simulink model "RT_01"  (R2018b)
settings: Solver=FixedStepAuto  StartTime=0.0  StopTime=40  FixedStep=0.01  RelTol=1e-3
undefined symbols (not defined in the file): circle, DiscIntNeverNeededParam, Measurement_Computing, National_Instruments, PCI, QUAD04
libraries: sldrtlib x25, simulink x8, simulink_extras x2
(part 2 of 2)

== matlab function RT_01/Set point/Path Planning Circle/Inverse Kinematics JS1 ==
  data: EE_r input; P output; solution input
function P  = IK_JS(EE_r,solution)
a1=75; a2=270; a3=90; d1=335; d4=295; d7=80;
l = size(EE_r,1);   % Số điểm cần tính động học nghịch khi quy hoạch đường đi
emt1 = zeros(l,13); % Mảng rỗng để chứa ngõ t, the(t), v(t)
for n=1:l           % Vòng for tính động học nghịch từng điểm
    emt = zeros(8,6);
    m = 0;
    px =    EE_r(n,2);
    py =    EE_r(n,3);
    pz =    EE_r(n,4);
    roll =  EE_r(n,5);  
    pitch = EE_r(n,6);
    yaw =   EE_r(n,7);
    r11 = cos(yaw)*cos(pitch);
    r21 = sin(yaw)*cos(pitch);
    r31 = -sin(pitch);
    r12 = cos(yaw)*sin(pitch)*sin(roll) - sin(yaw)*cos(roll);
    r22 = sin(yaw)*sin(pitch)*sin(roll) + cos(yaw)*cos(roll);
    r32 = cos(pitch)*sin(roll);
    r13 = cos(yaw)*sin(pitch)*cos(roll) + sin(yaw)*sin(roll);
    r23 = sin(yaw)*sin(pitch)*cos(roll) - cos(yaw)*sin(roll);
    r33 = cos(pitch)*cos(roll);
    % Find the1
    a_1 = py - r23*d7;
    b_1 = - px + r13*d7;
    d_1 = 0;
    the11 = basic_01(a_1,b_1,d_1);

    for i = 1:2
        % Find the2
        u = cos(the11(i))*(px-d7*r13) + sin(the11(i))*(py-r23*d7) - a1;
        v = pz - d1 - r33*d7;
        a_2 = v;
        b_2 = u;
        d_2 = (a3^2+d4^2-u^2-v^2-a2^2)/(-2*a2);
        if a_2*a_2 + b_2*b_2 - d_2*d_2 >=0
            the22 = basic_01(a_2,b_2,d_2);
        else
            continue;
        end

        for j = 1:2
            % Find the3
            a_3 = a3;
            b_3 = d4;
            c_3 = u*sin(the22(j)) + v*cos(the22(j)) - a2;
            d_3 = u*cos(the22(j)) - v*sin(the22(j));
            the33 = basic_02(a_3,b_3,c_3,d_3);

            % Find the5
            c5 = (r13*cos(the11(i))*cos(the22(j)) - r33*sin(the22(j)) + r23*cos(the22(j))*sin(the11(i)))*cos(the33) - (r33*cos(the22(j)) + r13*cos(the11(i))*sin(the22(j)) + r23*sin(the11(i))*sin(the22(j)))*sin(the33);
            if 1*1 + 0*0 - c5*c5 >=0
                the55 = basic_01(1,0,c5);
            else
                continue;
            end
            for k = 1:2
                % Find the4
                m = m+1;
                s4 = (r23*cos(the11(i)) - r13*sin(the11(i)))/(sin(the55(k)));
                c4 = (r33*cos(the22(j)) + r13*cos(the11(i))*sin(the22(j)) + r23*sin(the11(i))*sin(the22(j)) + sin(the33)*cos(the55(k))) / (-cos(the33)*sin(the55(k)));
                the44 = atan2(s4,c4);

                % Find the6
                a_6 = r21*cos(the11(i)) - r11*sin(the11(i));
                b_6 = r22*cos(the11(i)) - r12*sin(the11(i));
                c_6 = -sin(the44)*cos(the55(k));
                d_6 = cos(the44);
                the66 = basic_02(a_6,b_6,c_6,-d_6);
                emt(m,:)=[the11(i),the22(j),the33,the44,the55(k),the66];
            end
        end
    end
    % the = emt(solution,:);
    the1 = emt(solution,1);
    the2 = emt(solution,2);
    the3 = emt(solution,3);
    the4 = emt(solution,4);
    the5 = emt(solution,5);
    the6 = emt(solution,6);
%     the_r = [the1;the2;the3;the4;the5;the6];
%     emt1(n,:) = [(n-1)*t/l,the1,the2,the3,the4,the5,the6,0,0,0,0,0,0];
    emt1(n,:) = [EE_r(n,1),the1,the2,the3,the4,the5,the6,0,0,0,0,0,0];
end
P=emt1;
end

function x = basic_01(a, b, d) % a*cos(x) + b*sin(x) = d
    anp = atan2(b, a);
    
    x1 = anp + atan2(sqrt(a*a + b*b - d*d), d);
    x2 = anp + atan2(-sqrt(a*a + b*b - d*d), d);
    x = [x1; x2];
end   

function x = basic_02(a, b, c, d) 
    % a*cos(x) - b*sin(x) = c
    % b*cos(x) + a*sin(x) = d
    sin = (d - b*c/a) / (b^2/a + a);
    cos = (c + b*d/a) / (b^2/a + a);
    x = atan2(sin,cos);
end

== matlab function RT_01/Set point/Path Planning Circle/Circle CS ==
  data: clock input; EE_r output
function EE_r = TP_Circle(clock)
% H=ScopeData.signals.values(:,1:3);
t = clock-10;
f=0.1; %hz
Px_r = 450;
Py_r = 0+100*sin(2*pi*f*t);
Pz_r = 550+100*cos(2*pi*f*t);
% roll_r=pi/3;
% pitch_r=pi/6;
% yaw_r=pi/2;
roll_r = 0*pi/2;
pitch_r = -pi/2;
yaw_r = pi;
EE_r = [Px_r,Py_r,Pz_r,roll_r,pitch_r,yaw_r]';

== matlab function RT_01/Set point/Path Planning Circle/Trajectory Planning CS ==
  data: clock input; EE_r output; P input
function EE_r = TP_CS_6DOF(clock,P)
t=clock;
% H=ScopeData.signals.values(:,1:3); Lưu data để sử dụng spline
%% Quy hoạch quỹ đạo
k = size(P,1)-1;                    % Số giai đoạn chạy, i điểm thì i-1 giai đoạn
ai = zeros(k,24);                    % Ma trận K*8 lưu các giá trị a0 - a4 của X, Y
for i=1:k
    ai(i,:) = TP_CS(P(i,:),P(i+1,:));  % Tính giá trị a0 - a4 đối với từng điểm P(x,y)
end
%% Xuất quỹ đạo
% P0 = [ti; q0x; q0y; q0z; q0roll; q0pitch; q0yaw; v0x; v0y; v0z; v0roll; v0pitch; v0yaw]
% Pf = [tf; qfx; qfy; qfz; qfroll; qfpitch; qfyaw; vfx; vfy; vfz; vfroll; vfpitch; vfyaw]
ti = P(2,1);                        % Thời gian lấy mẫu giữa 2 điểm
if (t<P(k+1,1))
    j = floor(t/ti) + 1;            % Xác định giai đoạn hiện tại của quỹ đạo
    Px    =  ai(j,1) +  ai(j,2)*t +  ai(j,3)*t^2 + ai(j,4)*t^3;
    Py    =  ai(j,5) +  ai(j,6)*t +  ai(j,7)*t^2 + ai(j,8)*t^3;
    Pz    =  ai(j,9) + ai(j,10)*t + ai(j,11)*t^2 + ai(j,12)*t^3;
    roll  = ai(j,13) + ai(j,14)*t + ai(j,15)*t^2 + ai(j,16)*t^3;
    pitch = ai(j,17) + ai(j,18)*t + ai(j,19)*t^2 + ai(j,20)*t^3;
    yaw   = ai(j,21) + ai(j,22)*t + ai(j,23)*t^2 + ai(j,24)*t^3;
else
    Px    = P(k+1,2);
    Py    = P(k+1,3);
    Pz    = P(k+1,4);
    roll  = P(k+1,5);
    pitch = P(k+1,6);
    yaw   = P(k+1,7);
end
EE_r = [Px,Py,Pz,roll,pitch,yaw]';
end

function C = TP_CS(P0,Pf)
% 0x: điểm đầu phương X, fx: điểm cuối phương X
% 0y: điểm đầu phương Y, fy: điểm cuối phương Y
% 0z: điểm đầu phương Y, fz: điểm cuối phương Y
% 0roll:  hướng roll đầu, froll: hướng roll cuối
% 0pitch: điểm pitch đầu, fpitch: hướng pitch cuối
% 0yaw:     điểm yaw đầu, fyaw: hướng yaw cuối
% P0 = [ti; q0x; q0y; q0z; q0roll; q0pitch; q0yaw; v0x; v0y; v0z; v0roll; v0pitch; v0yaw]
% Pf = [tf; qfx; qfy; qfz; qfroll; qfpitch; qfyaw; vfx; vfy; vfz; vfroll; vfpitch; vfyaw]
% Phương trình quy hoạch quỹ đạo bậc 3: q = a0 + a1*t + a2*t^2 + a3*t^3
t0 = P0(1);
tf = Pf(1);
A = [1   t0   t0^2   t0^3;     % q0
     0   1    2*t0   3*t0^2;   % v0
     1   tf   tf^2   tf^3;     % qf
     0   1    2*tf   3*tf^2];  % vf
  
Bx     = [P0(2);  0;  Pf(2); 0];   % [    q0x     v0x     qfx     vfx]
By     = [P0(3);  0;  Pf(3); 0];   % [    q0y     v0y     qfy     vfy]
Bz     = [P0(4);  0;  Pf(4); 0];   % [    q0z     v0z     qfz     vfz]
Broll  = [P0(5);  0;  Pf(5); 0];   % [ q0roll  v0roll  qfroll  vfroll]
Bpitch = [P0(6);  0;  Pf(6); 0];   % [q0pitch v0pitch qfpitch vfpitch]
Byaw   = [P0(7);  0;  Pf(7); 0];   % [  q0yaw   v0yaw   qfyaw   vfyaw]

Cx     = A\Bx;
Cy     = A\By;
Cz     = A\Bz;
Croll  = A\Broll;
Cpitch = A\Bpitch;
Cyaw   = A\Byaw;
C = [    Cx(1),     Cx(2),     Cx(3),     Cx(4),...   % [    a0x     a1x     a2x     a3x]
         Cy(1),     Cy(2),     Cy(3),     Cy(4),...   % [    a0y     a1y     a2y     a3y]
         Cz(1),     Cz(2),     Cz(3),     Cz(4),...   % [    a0z     a1z     a2z     a3z]
      Croll(1),  Croll(2),  Croll(3),  Croll(4),...   % [ a0roll  a1roll  a2roll  a3roll]
     Cpitch(1), Cpitch(2), Cpitch(3), Cpitch(4),...   % [a0pitch a1pitch a2pitch a3pitch]
       Cyaw(1),   Cyaw(2),   Cyaw(3),   Cyaw(4)];     % [  a0yaw   a1yaw   a2yaw   a3yaw]
end

== matlab function RT_01/Set point/Path Planning Circle/Trajectory Planning JS ==
  data: t input; the_r output; P input
function the_r = TP_JS_6DOF(t,P)
% H=ScopeData.signals.values(:,1:3); Lưu data để sử dụng spline
%% Quy hoạch quỹ đạo
k = size(P,1)-1;                    % Số giai đoạn chạy, i điểm thì i-1 giai đoạn
ai = zeros(k,24);                    % Ma trận K*8 lưu các giá trị a0 - a4 của X, Y
for i=1:k
    ai(i,:) = TP_JS(P(i,:),P(i+1,:));  % Tính giá trị a0 - a4 đối với từng điểm P(x,y)
end
%% Xuất quỹ đạo
% the0 = [ti; q01; q02; q03; q04; q05; q06; v01; v02; v03; v04; v05; v06]
% thef = [tf; qf1; qf2; qf3; q04; q05; q06; vf1; v02; v03; v04; v05; v06]
ti = P(2,1);                        % Thời gian lấy mẫu giữa 2 điểm
if (t<P(k+1,1))
    j = floor(t/ti) + 1;            % Xác định giai đoạn hiện tại của quỹ đạo
    the1 = ai(j,1)  + ai(j,2)*t  + ai(j,3)*t^2  + ai(j,4)*t^3;
    the2 = ai(j,5)  + ai(j,6)*t  + ai(j,7)*t^2  + ai(j,8)*t^3;
    the3 = ai(j,9)  + ai(j,10)*t + ai(j,11)*t^2 + ai(j,12)*t^3;
    the4 = ai(j,13) + ai(j,14)*t + ai(j,15)*t^2 + ai(j,16)*t^3;
    the5 = ai(j,17) + ai(j,18)*t + ai(j,19)*t^2 + ai(j,20)*t^3;
    the6 = ai(j,21) + ai(j,22)*t + ai(j,23)*t^2 + ai(j,24)*t^3;
else
    the1 = P(k+1,2);
    the2 = P(k+1,3);
    the3 = P(k+1,4);
    the4 = P(k+1,5);
    the5 = P(k+1,6);
    the6 = P(k+1,7);
end
the_r = [the1,the2,the3,the4,the5,the6]';
end

function C = TP_JS(P0,Pf)
% 01: điểm đầu khớp 1, f1: điểm cuối khớp 1
% 02: điểm đầu khớp 2, f2: điểm cuối khớp 2
% 03: điểm đầu khớp 3, f3: điểm cuối khớp 3
% 04: điểm đầu khớp 4, f4: điểm cuối khớp 4
% 05: điểm đầu khớp 5, f5: điểm cuối khớp 5
% 06: điểm đầu khớp 6, f6: điểm cuối khớp 6
% the0 = [ti; q01; q02; q03; q04; q05; q06; v01; v02; v03; v04; v05; v06]
% thef = [tf; qf1; qf2; qf3; q04; q05; q06; vf1; v02; v03; v04; v05; v06]
% Phương trình quy hoạch quỹ đạo bậc 3: q = a0 + a1*t + a2*t^2 + a3*t^3
t0 = P0(1);
tf = Pf(1);
A = [1   t0   t0^2   t0^3;     % q0
     0   1    2*t0   3*t0^2;   % v0
     1   tf   tf^2   tf^3;     % qf
     0   1    2*tf   3*tf^2];  % vf
  
B1 = [P0(2);   P0(8);  Pf(2);  Pf(8)];  % [q01 v01 qf1 vf1]
B2 = [P0(3);   P0(9);  Pf(3);  Pf(9)];  % [q02 v02 qf2 vf2]
B3 = [P0(4);  P0(10);  Pf(4); Pf(10)];  % [q03 v03 qf3 vf3]
B4 = [P0(5);  P0(11);  Pf(5); Pf(11)];  % [q04 v04 qf4 vf4]
B5 = [P0(6);  P0(12);  Pf(6); Pf(12)];  % [q05 v05 qf5 vf5]
B6 = [P0(7);  P0(13);  Pf(7); Pf(13)];  % [q06 v06 qf6 vf6]

C1 = A\B1;
C2 = A\B2;
C3 = A\B3;
C4 = A\B4;
C5 = A\B5;
C6 = A\B6;

C = [C1(1), C1(2),  C1(3),  C1(4),...   % [a01 a11 a21 a31]
     C2(1), C2(2),  C2(3),  C2(4),...   % [a02 a12 a22 a32]
     C3(1), C3(2),  C3(3),  C3(4),...   % [a03 a13 a23 a33]
     C4(1), C4(2),  C4(3),  C4(4),...   % [a04 a14 a24 a34]
     C5(1), C5(2),  C5(3),  C5(4),...   % [a05 a15 a25 a35]
     C6(1), C6(2),  C6(3),  C6(4)];     % [a06 a16 a26 a36]
end

== matlab function RT_01/Set point/Path Planning Circle/Inverse Kinematics JS ==
  data: EE_r input; P output; solution input
function P  = IK_JS(EE_r,solution)
a1=75; a2=270; a3=90; d1=335; d4=295; d7=80;
l = size(EE_r,1);   % Số điểm cần tính động học nghịch khi quy hoạch đường đi
emt1 = zeros(l,13); % Mảng rỗng để chứa ngõ t, the(t), v(t)
for n=1:l           % Vòng for tính động học nghịch từng điểm
    emt = zeros(8,6);
    m = 0;
    px =    EE_r(n,2);
    py =    EE_r(n,3);
    pz =    EE_r(n,4);
    roll =  EE_r(n,5);  
    pitch = EE_r(n,6);
    yaw =   EE_r(n,7);
    r11 = cos(yaw)*cos(pitch);
    r21 = sin(yaw)*cos(pitch);
    r31 = -sin(pitch);
    r12 = cos(yaw)*sin(pitch)*sin(roll) - sin(yaw)*cos(roll);
    r22 = sin(yaw)*sin(pitch)*sin(roll) + cos(yaw)*cos(roll);
    r32 = cos(pitch)*sin(roll);
    r13 = cos(yaw)*sin(pitch)*cos(roll) + sin(yaw)*sin(roll);
    r23 = sin(yaw)*sin(pitch)*cos(roll) - cos(yaw)*sin(roll);
    r33 = cos(pitch)*cos(roll);
    % Find the1
    a_1 = py - r23*d7;
    b_1 = - px + r13*d7;
    d_1 = 0;
    the11 = basic_01(a_1,b_1,d_1);

    for i = 1:2
        % Find the2
        u = cos(the11(i))*(px-d7*r13) + sin(the11(i))*(py-r23*d7) - a1;
        v = pz - d1 - r33*d7;
        a_2 = v;
        b_2 = u;
        d_2 = (a3^2+d4^2-u^2-v^2-a2^2)/(-2*a2);
        if a_2*a_2 + b_2*b_2 - d_2*d_2 >=0
            the22 = basic_01(a_2,b_2,d_2);
        else
            continue;
        end

        for j = 1:2
            % Find the3
            a_3 = a3;
            b_3 = d4;
            c_3 = u*sin(the22(j)) + v*cos(the22(j)) - a2;
            d_3 = u*cos(the22(j)) - v*sin(the22(j));
            the33 = basic_02(a_3,b_3,c_3,d_3);

            % Find the5
            c5 = (r13*cos(the11(i))*cos(the22(j)) - r33*sin(the22(j)) + r23*cos(the22(j))*sin(the11(i)))*cos(the33) - (r33*cos(the22(j)) + r13*cos(the11(i))*sin(the22(j)) + r23*sin(the11(i))*sin(the22(j)))*sin(the33);
            if 1*1 + 0*0 - c5*c5 >=0
                the55 = basic_01(1,0,c5);
            else
                continue;
            end
            for k = 1:2
                % Find the4
                m = m+1;
                s4 = (r23*cos(the11(i)) - r13*sin(the11(i)))/(sin(the55(k)));
                c4 = (r33*cos(the22(j)) + r13*cos(the11(i))*sin(the22(j)) + r23*sin(the11(i))*sin(the22(j)) + sin(the33)*cos(the55(k))) / (-cos(the33)*sin(the55(k)));
                the44 = atan2(s4,c4);

                % Find the6
                a_6 = r21*cos(the11(i)) - r11*sin(the11(i));
                b_6 = r22*cos(the11(i)) - r12*sin(the11(i));
                c_6 = -sin(the44)*cos(the55(k));
                d_6 = cos(the44);
                the66 = basic_02(a_6,b_6,c_6,-d_6);
                emt(m,:)=[the11(i),the22(j),the33,the44,the55(k),the66];
            end
        end
    end
    % the = emt(solution,:);
    the1 = emt(solution,1);
    the2 = emt(solution,2);
    the3 = emt(solution,3);
    the4 = emt(solution,4);
    the5 = emt(solution,5);
    the6 = emt(solution,6);
%     the_r = [the1;the2;the3;the4;the5;the6];
%     emt1(n,:) = [(n-1)*t/l,the1,the2,the3,the4,the5,the6,0,0,0,0,0,0];
    emt1(n,:) = [EE_r(n,1),the1,the2,the3,the4,the5,the6,0,0,0,0,0,0];
end
P=emt1;
end

function x = basic_01(a, b, d) % a*cos(x) + b*sin(x) = d
    anp = atan2(b, a);
    
    x1 = anp + atan2(sqrt(a*a + b*b - d*d), d);
    x2 = anp + atan2(-sqrt(a*a + b*b - d*d), d);
    x = [x1; x2];
end   

function x = basic_02(a, b, c, d) 
    % a*cos(x) - b*sin(x) = c
    % b*cos(x) + a*sin(x) = d
    sin = (d - b*c/a) / (b^2/a + a);
    cos = (c + b*d/a) / (b^2/a + a);
    x = atan2(sin,cos);
end

== matlab function RT_01/Set point/Path Planning Circle/Trajectory Planning JS1 ==
  data: t input; the_r output; P input
function the_r = TP_JS_6DOF(t,P)
% H=ScopeData.signals.values(:,1:3); Lưu data để sử dụng spline
%% Quy hoạch quỹ đạo
k = size(P,1)-1;                    % Số giai đoạn chạy, i điểm thì i-1 giai đoạn
ai = zeros(k,24);                    % Ma trận K*8 lưu các giá trị a0 - a4 của X, Y
for i=1:k
    ai(i,:) = TP_JS(P(i,:),P(i+1,:));  % Tính giá trị a0 - a4 đối với từng điểm P(x,y)
end
%% Xuất quỹ đạo
% the0 = [ti; q01; q02; q03; q04; q05; q06; v01; v02; v03; v04; v05; v06]
% thef = [tf; qf1; qf2; qf3; q04; q05; q06; vf1; v02; v03; v04; v05; v06]
ti = P(2,1);                        % Thời gian lấy mẫu giữa 2 điểm
if (t<P(k+1,1))
    j = floor(t/ti) + 1;            % Xác định giai đoạn hiện tại của quỹ đạo
    the1 = ai(j,1)  + ai(j,2)*t  + ai(j,3)*t^2  + ai(j,4)*t^3;
    the2 = ai(j,5)  + ai(j,6)*t  + ai(j,7)*t^2  + ai(j,8)*t^3;
    the3 = ai(j,9)  + ai(j,10)*t + ai(j,11)*t^2 + ai(j,12)*t^3;
    the4 = ai(j,13) + ai(j,14)*t + ai(j,15)*t^2 + ai(j,16)*t^3;
    the5 = ai(j,17) + ai(j,18)*t + ai(j,19)*t^2 + ai(j,20)*t^3;
    the6 = ai(j,21) + ai(j,22)*t + ai(j,23)*t^2 + ai(j,24)*t^3;
else
    the1 = P(k+1,2);
    the2 = P(k+1,3);
    the3 = P(k+1,4);
    the4 = P(k+1,5);
    the5 = P(k+1,6);
    the6 = P(k+1,7);
end
the_r = [the1,the2,the3,the4,the5,the6]';
end

function C = TP_JS(P0,Pf)
% 01: điểm đầu khớp 1, f1: điểm cuối khớp 1
% 02: điểm đầu khớp 2, f2: điểm cuối khớp 2
% 03: điểm đầu khớp 3, f3: điểm cuối khớp 3
% 04: điểm đầu khớp 4, f4: điểm cuối khớp 4
% 05: điểm đầu khớp 5, f5: điểm cuối khớp 5
% 06: điểm đầu khớp 6, f6: điểm cuối khớp 6
% the0 = [ti; q01; q02; q03; q04; q05; q06; v01; v02; v03; v04; v05; v06]
% thef = [tf; qf1; qf2; qf3; q04; q05; q06; vf1; v02; v03; v04; v05; v06]
% Phương trình quy hoạch quỹ đạo bậc 3: q = a0 + a1*t + a2*t^2 + a3*t^3
t0 = P0(1);
tf = Pf(1);
A = [1   t0   t0^2   t0^3;     % q0
     0   1    2*t0   3*t0^2;   % v0
     1   tf   tf^2   tf^3;     % qf
     0   1    2*tf   3*tf^2];  % vf
  
B1 = [P0(2);   P0(8);  Pf(2);  Pf(8)];  % [q01 v01 qf1 vf1]
B2 = [P0(3);   P0(9);  Pf(3);  Pf(9)];  % [q02 v02 qf2 vf2]
B3 = [P0(4);  P0(10);  Pf(4); Pf(10)];  % [q03 v03 qf3 vf3]
B4 = [P0(5);  P0(11);  Pf(5); Pf(11)];  % [q04 v04 qf4 vf4]
B5 = [P0(6);  P0(12);  Pf(6); Pf(12)];  % [q05 v05 qf5 vf5]
B6 = [P0(7);  P0(13);  Pf(7); Pf(13)];  % [q06 v06 qf6 vf6]

C1 = A\B1;
C2 = A\B2;
C3 = A\B3;
C4 = A\B4;
C5 = A\B5;
C6 = A\B6;

C = [C1(1), C1(2),  C1(3),  C1(4),...   % [a01 a11 a21 a31]
     C2(1), C2(2),  C2(3),  C2(4),...   % [a02 a12 a22 a32]
     C3(1), C3(2),  C3(3),  C3(4),...   % [a03 a13 a23 a33]
     C4(1), C4(2),  C4(3),  C4(4),...   % [a04 a14 a24 a34]
     C5(1), C5(2),  C5(3),  C5(4),...   % [a05 a15 a25 a35]
     C6(1), C6(2),  C6(3),  C6(4)];     % [a06 a16 a26 a36]
end

== matlab function RT_01/Set point/Path Planning Circle/MATLAB Function ==
  data: clock input; y output
function y = Planning(clock)
if (clock < 5)
    y = 1;
elseif (clock >= 5) && (clock < 10)
    y = 2;
elseif (clock >= 10) && (clock < 30)
    y = 3;
elseif (clock >= 30) && (clock < 35)
    y = 4;
elseif (clock >= 35)
    y = 5;
else
    y = 5;
end
end

== matlab function RT_01/MATLAB Function3 ==
  data: the input; EE output
function EE  = FK_6DOF(the)
the1 = the(1);
the2 = the(2);
the3 = the(3);
the4 = the(4);
the5 = the(5);
the6 = the(6);
a1=75; a2=270; a3=90; d1=335; d4=295; d7=80;

T_0_EE = ...
[ cos(the6)*(cos(the5)*sin(the1)*sin(the4) + cos(the2 + the3)*cos(the1)*sin(the5) + cos(the1)*cos(the2)*cos(the4)*cos(the5)*sin(the3) + cos(the1)*cos(the3)*cos(the4)*cos(the5)*sin(the2)) - sin(the6)*(cos(the1)*cos(the2)*sin(the3)*sin(the4) - cos(the4)*sin(the1) + cos(the1)*cos(the3)*sin(the2)*sin(the4)), - cos(the6)*(cos(the1)*cos(the2)*sin(the3)*sin(the4) - cos(the4)*sin(the1) + cos(the1)*cos(the3)*sin(the2)*sin(the4)) - sin(the6)*(cos(the5)*sin(the1)*sin(the4) + cos(the2 + the3)*cos(the1)*sin(the5) + cos(the1)*cos(the2)*cos(the4)*cos(the5)*sin(the3) + cos(the1)*cos(the3)*cos(the4)*cos(the5)*sin(the2)), cos(the2 + the3)*cos(the1)*cos(the5) - sin(the5)*(sin(the1)*sin(the4) + cos(the1)*cos(the2)*cos(the4)*sin(the3) + cos(the1)*cos(the3)*cos(the4)*sin(the2)), a1*cos(the1) + a2*cos(the1)*sin(the2) + d4*cos(the1)*cos(the2)*cos(the3) + a3*cos(the1)*cos(the2)*sin(the3) + a3*cos(the1)*cos(the3)*sin(the2) - d4*cos(the1)*sin(the2)*sin(the3) - d7*sin(the1)*sin(the4)*sin(the5) + d7*cos(the1)*cos(the2)*cos(the3)*cos(the5) - d7*cos(the1)*cos(the5)*sin(the2)*sin(the3) - d7*cos(the1)*cos(the2)*cos(the4)*sin(the3)*sin(the5) - d7*cos(the1)*cos(the3)*cos(the4)*sin(the2)*sin(the5);
  cos(the6)*(cos(the2 + the3)*sin(the1)*sin(the5) - cos(the1)*cos(the5)*sin(the4) + cos(the2)*cos(the4)*cos(the5)*sin(the1)*sin(the3) + cos(the3)*cos(the4)*cos(the5)*sin(the1)*sin(the2)) - sin(the6)*(cos(the1)*cos(the4) + cos(the2)*sin(the1)*sin(the3)*sin(the4) + cos(the3)*sin(the1)*sin(the2)*sin(the4)), - cos(the6)*(cos(the1)*cos(the4) + cos(the2)*sin(the1)*sin(the3)*sin(the4) + cos(the3)*sin(the1)*sin(the2)*sin(the4)) - sin(the6)*(cos(the2 + the3)*sin(the1)*sin(the5) - cos(the1)*cos(the5)*sin(the4) + cos(the2)*cos(the4)*cos(the5)*sin(the1)*sin(the3) + cos(the3)*cos(the4)*cos(the5)*sin(the1)*sin(the2)), cos(the2 + the3)*cos(the5)*sin(the1) - sin(the5)*(cos(the2)*cos(the4)*sin(the1)*sin(the3) - cos(the1)*sin(the4) + cos(the3)*cos(the4)*sin(the1)*sin(the2)), a1*sin(the1) + a2*sin(the1)*sin(the2) + d4*cos(the2)*cos(the3)*sin(the1) + a3*cos(the2)*sin(the1)*sin(the3) + a3*cos(the3)*sin(the1)*sin(the2) + d7*cos(the1)*sin(the4)*sin(the5) - d4*sin(the1)*sin(the2)*sin(the3) + d7*cos(the2)*cos(the3)*cos(the5)*sin(the1) - d7*cos(the5)*sin(the1)*sin(the2)*sin(the3) - d7*cos(the2)*cos(the4)*sin(the1)*sin(the3)*sin(the5) - d7*cos(the3)*cos(the4)*sin(the1)*sin(the2)*sin(the5);
                                                                                                                                                                                          - cos(the6)*(sin(the2 + the3)*sin(the5) - cos(the2 + the3)*cos(the4)*cos(the5)) - cos(the2 + the3)*sin(the4)*sin(the6),                                                                                                                                                                                             sin(the6)*(sin(the2 + the3)*sin(the5) - cos(the2 + the3)*cos(the4)*cos(the5)) - cos(the2 + the3)*cos(the6)*sin(the4),                                                                                        - sin(the2 + the3)*cos(the5) - cos(the2 + the3)*cos(the4)*sin(the5),                                                                                                                                        d1 + a2*cos(the2) + a3*cos(the2)*cos(the3) - d4*cos(the2)*sin(the3) - d4*cos(the3)*sin(the2) - a3*sin(the2)*sin(the3) - d7*cos(the2)*cos(the5)*sin(the3) - d7*cos(the3)*cos(the5)*sin(the2) - d7*cos(the2)*cos(the3)*cos(the4)*sin(the5) + d7*cos(the4)*sin(the2)*sin(the3)*sin(the5);
                                                                                                                                                                                                                                                                                                               0,                                                                                                                                                                                                                                                                                                                0,                                                                                                                                                          0,                                                                                                                                                                                                                                                                                                                                                                                                                            1];
 
r11 = T_0_EE(1,1);
r21 = T_0_EE(2,1);
r31 = T_0_EE(3,1);
r12 = T_0_EE(1,2);
r22 = T_0_EE(2,2);
r32 = T_0_EE(3,2);
r13 = T_0_EE(1,3);
r23 = T_0_EE(2,3);
r33 = T_0_EE(3,3);
pitch = atan2(-r31,sqrt(r11^2+r21^2));
if pitch == pi/2
    yaw = 0;
    roll = atan2(r12,r22);
elseif pitch == -pi/2
    yaw = 0;
    roll = -atan2(r12,r22) ;     
else
    yaw = atan2(r21/cos(pitch),r11/cos(pitch));
    roll = atan2(r32/cos(pitch),r33/cos(pitch));
end
Px = T_0_EE(1,4);
Py = T_0_EE(2,4);
Pz = T_0_EE(3,4);
EE = [Px,Py,Pz,roll,pitch,yaw];
